simulink model "InvertedPendulumSSTest"  (Simulink 7.7)
settings: Solver=ode5  StartTime=0.0  StopTime=10  FixedStep=.0005  RelTol=1e-3
PreLoadFcn:
  | StateSpacePrelimv2
values from neighbouring files (symbols this model uses):
  ba = 6.5E-6    (= 6.5e-06)    [StateSpacePrelimv2.m]
  btf = 1.08586e-5    (= 1.08586e-05)    [StateSpacePrelimv2.m]
  btr = 4.8593e-5    (= 4.8593e-05)    [StateSpacePrelimv2.m]
  CONTROLLER_SWITCH_POINT = .30    (= 0.3)    [StateSpacePrelimv2.m]
  g = 9.81    [StateSpacePrelimv2.m]
  I1zt = 6.78e-4 + 3.50514e-5    (= 0.0007130514)    [StateSpacePrelimv2.m]
  Ix2 = 8.1e-6    (= 8.1e-06)    [StateSpacePrelimv2.m]
  Ixz2 = 2.03e-5    (= 2.03e-05)    [StateSpacePrelimv2.m]
  Iy2 = 3.711e-4    (= 0.0003711)    [StateSpacePrelimv2.m]
  Iz2 = 3.646e-4    (= 0.0003646)    [StateSpacePrelimv2.m]
  K = lqr(A,B,Q,R)    [StateSpacePrelimv2.m]
  Ka = 1    [StateSpacePrelimv2.m]
  Kb = 0.04    [StateSpacePrelimv2.m]
  Kt = 0.0314499    [StateSpacePrelimv2.m]
  l1 = 0.10825640    (= 0.1082564)    [StateSpacePrelimv2.m]
  l2c = 0.0856786    [StateSpacePrelimv2.m]
  m2 = 0.0820142    [StateSpacePrelimv2.m]
  Rm = 1.85    [StateSpacePrelimv2.m]
  tau = .01    (= 0.01)    [StateSpacePrelimv2.m]
  Tca = 7e-6    (= 7e-06)    [StateSpacePrelimv2.m]
  Tctf = 0.022439    [StateSpacePrelimv2.m]
  Tctr = 0.0143096    [StateSpacePrelimv2.m]
  Vsupply = 24    [StateSpacePrelimv2.m]
settings Model: Creator=gshiva  LastModifiedBy=jrpeterson

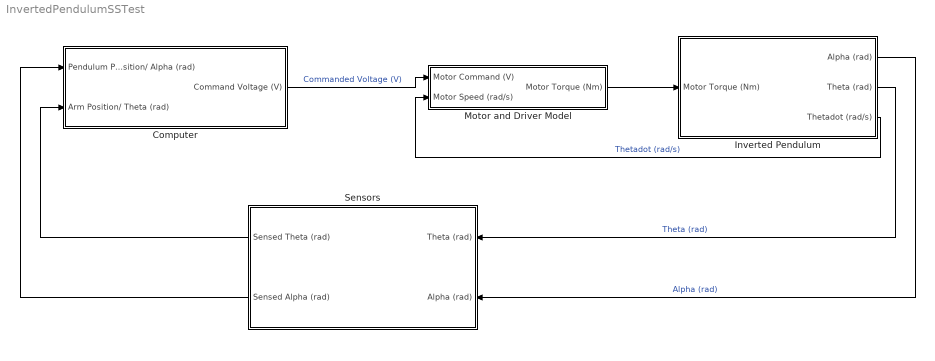
== system InvertedPendulumSSTest ==
  Computer : Subsystem
  Inverted Pendulum : Subsystem
  Motor and Driver Model : Subsystem
  Sensors : Subsystem
  wires:
  Computer/1(Command Voltage (V)) -> Motor and Driver Model/1(Motor Command (V))  "Commanded Voltage (V)"
  Sensors/2(Sensed Alpha (rad)) -> Computer/1(Pendulum Position/ Alpha (rad))
  Sensors/1(Sensed Theta (rad)) -> Computer/2(Arm Position/ Theta (rad))
  Inverted Pendulum/2(Theta (rad)) -> Sensors/1(Theta (rad))  "Theta (rad)"
  Inverted Pendulum/1(Alpha (rad)) -> Sensors/2(Alpha (rad))  "Alpha (rad)"
  Motor and Driver Model/1(Motor Torque (Nm)) -> Inverted Pendulum/1(Motor Torque (Nm))
  Inverted Pendulum/3(Thetadot (rad/s)) -> Motor and Driver Model/2(Motor Speed (rad/s))  "Thetadot (rad/s)"

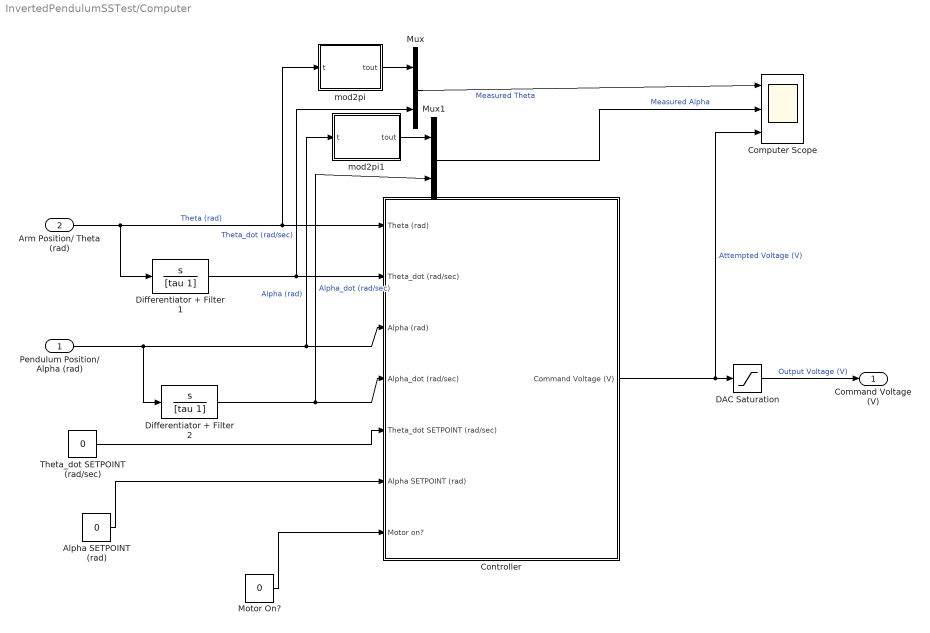
== system InvertedPendulumSSTest/Computer ==
  Pendulum Position/ Alpha (rad) : Inport
  Arm Position/ Theta (rad) : Inport  Port=2
  Alpha SETPOINT (rad) : Constant  Value=0
  Computer Scope : Scope  NumInputPorts=3
      settings: YMin=-10~-25~-800000  YMax=17.5~325~900000  SaveName=ScopeData3
  Controller : Subsystem
  DAC Saturation : Saturate  UpperLimit=10  LowerLimit=-10
  Differentiator + Filter 1 : TransferFcn  Numerator=[1 0]  Denominator=[tau 1]
  Differentiator + Filter 2 : TransferFcn  Numerator=[1 0]  Denominator=[tau 1]
  Motor On? : Constant  Value=0
  Mux : Mux  Inputs=2
  Mux1 : Mux  Inputs=2
  Theta_dot SETPOINT (rad/sec) : Constant  Value=0
  mod2pi : Stateflow chart  TreatAsAtomicUnit=on
  mod2pi1 : Stateflow chart  TreatAsAtomicUnit=on
  Command Voltage (V) : Outport
  wires:
  DAC Saturation/1 -> Command Voltage (V)/1  "Output Voltage (V)"
  Arm Position/ Theta (rad)/1 -> Differentiator + Filter 1/1, Controller/1(Theta (rad)), mod2pi/1(t)  "Theta (rad)"
  Differentiator + Filter 1/1 -> Controller/2(Theta_dot (rad/sec)), Mux/2  "Theta_dot (rad/sec)"
  Pendulum Position/ Alpha (rad)/1 -> Differentiator + Filter 2/1, Controller/3(Alpha (rad)), mod2pi1/1(t)  "Alpha (rad)"
  Differentiator + Filter 2/1 -> Mux1/2, Controller/4(Alpha_dot (rad/sec))  "Alpha_dot (rad/sec)"
  Controller/1(Command Voltage (V)) -> DAC Saturation/1, Computer Scope/3  "Attempted Voltage (V)"
  Theta_dot SETPOINT (rad/sec)/1 -> Controller/5(Theta_dot SETPOINT (rad/sec))
  Alpha SETPOINT (rad)/1 -> Controller/6(Alpha SETPOINT (rad))
  Mux/1 -> Computer Scope/1  "Measured Theta"
  Mux1/1 -> Computer Scope/2  "Measured Alpha"
  Motor On?/1 -> Controller/7(Motor on?)
  mod2pi/1(tout) -> Mux/1
  mod2pi1/1(tout) -> Mux1/1

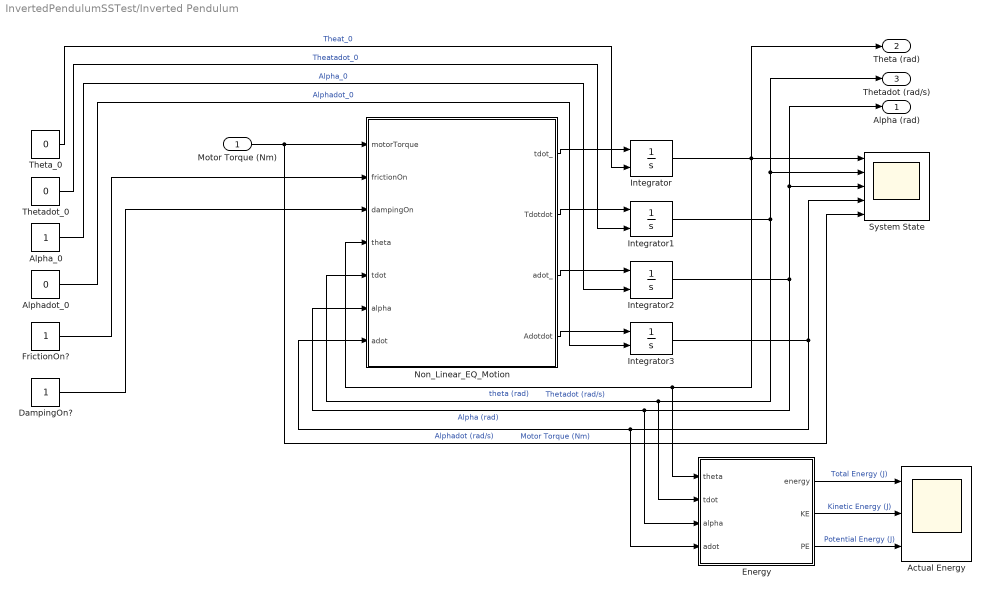
== system InvertedPendulumSSTest/Inverted Pendulum ==
  Motor Torque (Nm) : Inport
  Actual Energy : Scope  NumInputPorts=3
      settings: TimeRange=5  YMin=-0.07~0~-0.14  YMax=0.1~0.175~1.38778e-17  SaveName=Actual_Energy
  Alpha_0 : Constant
  Alphadot_0 : Constant  Value=0
  DampingOn? : Constant
  Energy : Stateflow chart  TreatAsAtomicUnit=on
  FrictionOn? : Constant
  Integrator{,1..3} (4 alike) : Integrator  InitialConditionSource=external
  Non_Linear_EQ_Motion : Stateflow chart  TreatAsAtomicUnit=on
  System State : Scope  NumInputPorts=5
      settings: TimeRange=10  YMin=-1~-20~0~-20~-0.4  YMax=4~20~5~20~0.4
  Theta_0 : Constant  Value=0
  Thetadot_0 : Constant  Value=0
  Alpha (rad) : Outport
  Theta (rad) : Outport  Port=2
  Thetadot (rad/s) : Outport  Port=3
  wires:
  Motor Torque (Nm)/1 -> Non_Linear_EQ_Motion/1(motorTorque), System State/5  "Motor Torque (Nm)"
  Non_Linear_EQ_Motion/1(tdot_) -> Integrator/1
  Theta_0/1 -> Integrator/2  "Theat_0"
  Non_Linear_EQ_Motion/2(Tdotdot) -> Integrator1/1
  Non_Linear_EQ_Motion/3(adot_) -> Integrator2/1
  Non_Linear_EQ_Motion/4(Adotdot) -> Integrator3/1
  Thetadot_0/1 -> Integrator1/2  "Theatadot_0"
  Alpha_0/1 -> Integrator2/2  "Alpha_0"
  Alphadot_0/1 -> Integrator3/2  "Alphadot_0"
  Integrator/1 -> System State/1, Theta (rad)/1, Non_Linear_EQ_Motion/4(theta), Energy/1(theta)  "theta (rad)"
  Integrator1/1 -> Non_Linear_EQ_Motion/5(tdot), Energy/2(tdot), System State/2, Thetadot (rad/s)/1  "Thetadot (rad/s)"
  Integrator2/1 -> System State/3, Alpha (rad)/1, Non_Linear_EQ_Motion/6(alpha), Energy/3(alpha)  "Alpha (rad)"
  Integrator3/1 -> System State/4, Non_Linear_EQ_Motion/7(adot), Energy/4(adot)  "Alphadot (rad/s)"
  Energy/1(energy) -> Actual Energy/1  "Total Energy (J)"
  Energy/2(KE) -> Actual Energy/2  "Kinetic Energy (J)"
  Energy/3(PE) -> Actual Energy/3  "Potential Energy (J)"
  FrictionOn?/1 -> Non_Linear_EQ_Motion/2(frictionOn)
  DampingOn?/1 -> Non_Linear_EQ_Motion/3(dampingOn)

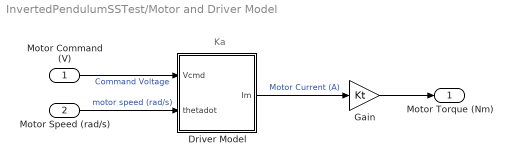
== system InvertedPendulumSSTest/Motor and Driver Model ==
  note: Ka
  Motor Command (V) : Inport
  Motor Speed (rad/s) : Inport  Port=2
  Driver Model : Stateflow chart  TreatAsAtomicUnit=on
  Gain : Gain  Gain=Kt
  Motor Torque (Nm) : Outport
  wires:
  Gain/1 -> Motor Torque (Nm)/1
  Driver Model/1(Im) -> Gain/1  "Motor Current (A)"
  Motor Command (V)/1 -> Driver Model/1(Vcmd)  "Command Voltage"
  Motor Speed (rad/s)/1 -> Driver Model/2(thetadot)  "motor speed (rad/s)"

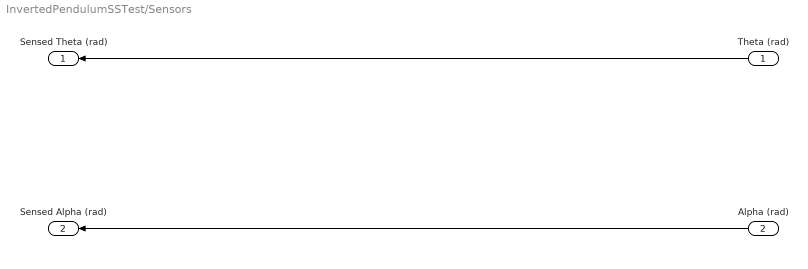
== system InvertedPendulumSSTest/Sensors ==
  Theta (rad) : Inport
  Alpha (rad) : Inport  Port=2
  Sensed Theta (rad) : Outport
  Sensed Alpha (rad) : Outport  Port=2
  wires:
  Alpha (rad)/1 -> Sensed Alpha (rad)/1
  Theta (rad)/1 -> Sensed Theta (rad)/1

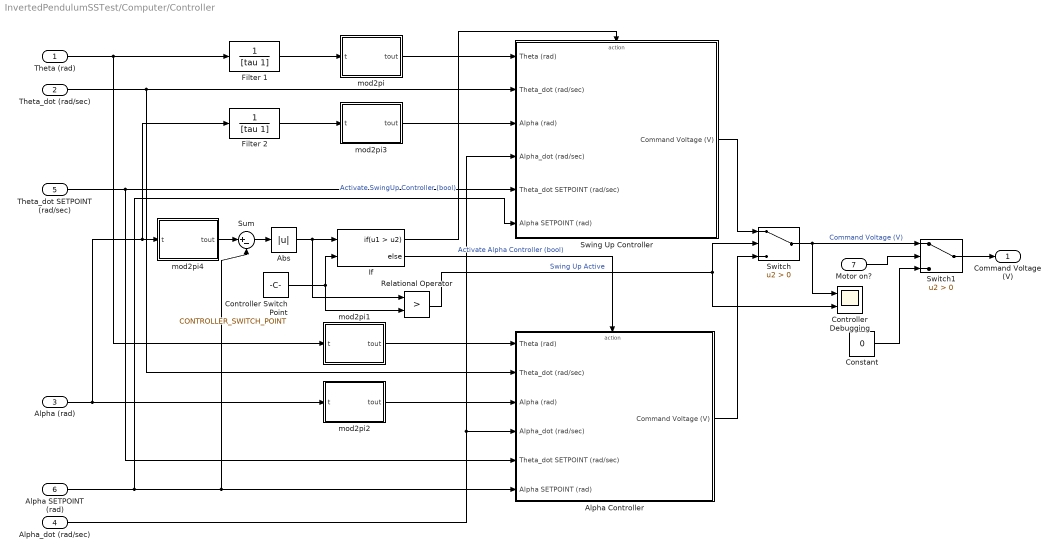
== system InvertedPendulumSSTest/Computer/Controller ==
  Theta (rad) : Inport
  Theta_dot (rad/sec) : Inport  Port=2
  Alpha (rad) : Inport  Port=3
  Alpha_dot (rad/sec) : Inport  Port=4
  Theta_dot SETPOINT (rad/sec) : Inport  Port=5
  Alpha SETPOINT (rad) : Inport  Port=6
  Motor on? : Inport  Port=7
  Abs : Abs
  Alpha Controller : Subsystem  TreatAsAtomicUnit=on
  Constant : Constant  Value=0
  Controller Debugging : Scope  NumInputPorts=2
      settings: YMin=-5~-5  YMax=5~5  SaveName=ScopeData2
  Controller Switch Point : Constant  Value=CONTROLLER_SWITCH_POINT
  Filter 1 : TransferFcn  Denominator=[tau 1]
  Filter 2 : TransferFcn  Denominator=[tau 1]
  If : If  NumInputs=2  IfExpression=u1 > u2
  Relational Operator : RelationalOperator  Operator=>  OutDataTypeStr=boolean
  Sum : Sum  Inputs=|+-
  Swing Up Controller : Subsystem  TreatAsAtomicUnit=on
  Switch : Switch  Criteria=u2 > Threshold
  Switch1 : Switch  Criteria=u2 > Threshold
  mod2pi : Stateflow chart  TreatAsAtomicUnit=on
  mod2pi1 : Stateflow chart  TreatAsAtomicUnit=on
  mod2pi2 : Stateflow chart  TreatAsAtomicUnit=on
  mod2pi3 : Stateflow chart  TreatAsAtomicUnit=on
  mod2pi4 : Stateflow chart  TreatAsAtomicUnit=on
  Command Voltage (V) : Outport
  wires:
  If/2 -> Alpha Controller/Action  "Activate Alpha Controller (bool)"
  Switch/1 -> Controller Debugging/1, Switch1/1  "Command Voltage (V)"
  If/1 -> Swing Up Controller/Action  "Activate SwingUp Controller (bool)"
  Controller Switch Point/1 -> If/2, Relational Operator/2
  Sum/1 -> Abs/1
  Alpha SETPOINT (rad)/1 -> Swing Up Controller/6(Alpha SETPOINT (rad)), Sum/2, Alpha Controller/6(Alpha SETPOINT (rad))
  Theta (rad)/1 -> mod2pi1/1(t), Filter 1/1
  Theta_dot (rad/sec)/1 -> Swing Up Controller/2(Theta_dot (rad/sec)), Alpha Controller/2(Theta_dot (rad/sec))
  Theta_dot SETPOINT (rad/sec)/1 -> Swing Up Controller/5(Theta_dot SETPOINT (rad/sec)), Alpha Controller/5(Theta_dot SETPOINT (rad/sec))
  Alpha_dot (rad/sec)/1 -> Swing Up Controller/4(Alpha_dot (rad/sec)), Alpha Controller/4(Alpha_dot (rad/sec))
  Alpha (rad)/1 -> Filter 2/1, mod2pi4/1(t), mod2pi2/1(t)
  Swing Up Controller/1(Command Voltage (V)) -> Switch/1
  Alpha Controller/1(Command Voltage (V)) -> Switch/3
  Relational Operator/1 -> Switch/2, Controller Debugging/2  "Swing Up Active"
  Switch1/1 -> Command Voltage (V)/1
  Constant/1 -> Switch1/3
  Motor on?/1 -> Switch1/2
  mod2pi/1(tout) -> Swing Up Controller/1(Theta (rad))
  mod2pi1/1(tout) -> Alpha Controller/1(Theta (rad))
  mod2pi2/1(tout) -> Alpha Controller/3(Alpha (rad))
  mod2pi3/1(tout) -> Swing Up Controller/3(Alpha (rad))
  Filter 1/1 -> mod2pi/1(t)
  Filter 2/1 -> mod2pi3/1(t)
  Abs/1 -> If/1, Relational Operator/1
  mod2pi4/1(tout) -> Sum/1

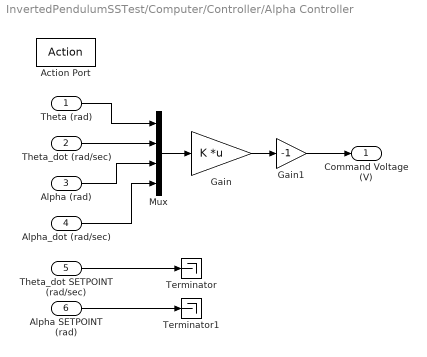
== system InvertedPendulumSSTest/Computer/Controller/Alpha Controller ==
  Theta (rad) : Inport
  Theta_dot (rad/sec) : Inport  Port=2
  Alpha (rad) : Inport  Port=3
  Alpha_dot (rad/sec) : Inport  Port=4
  Theta_dot SETPOINT (rad/sec) : Inport  Port=5
  Alpha SETPOINT (rad) : Inport  Port=6
  Action Port : ActionPort  ActionType=else
  Gain : Gain  Gain=K  Multiplication=Matrix(K*u)
  Gain1 : Gain  Gain=-1
  Mux : Mux
  Terminator : Terminator
  Terminator1 : Terminator
  Command Voltage (V) : Outport
  wires:
  Theta (rad)/1 -> Mux/1
  Theta_dot (rad/sec)/1 -> Mux/2
  Alpha (rad)/1 -> Mux/3
  Alpha_dot (rad/sec)/1 -> Mux/4
  Mux/1 -> Gain/1
  Gain/1 -> Gain1/1
  Gain1/1 -> Command Voltage (V)/1
  Theta_dot SETPOINT (rad/sec)/1 -> Terminator/1
  Alpha SETPOINT (rad)/1 -> Terminator1/1

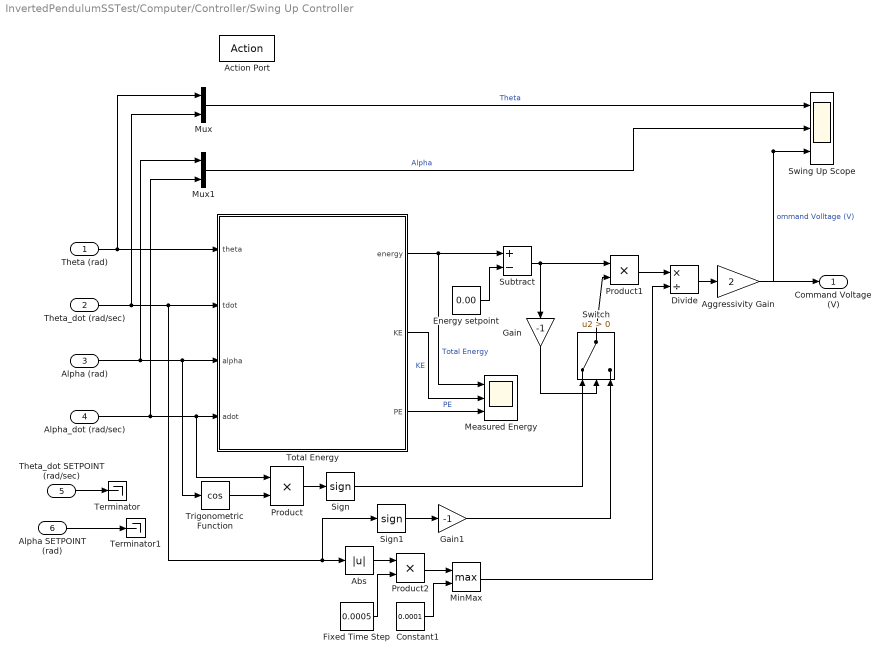
== system InvertedPendulumSSTest/Computer/Controller/Swing Up Controller ==
  Theta (rad) : Inport
  Theta_dot (rad/sec) : Inport  Port=2
  Alpha (rad) : Inport  Port=3
  Alpha_dot (rad/sec) : Inport  Port=4
  Theta_dot SETPOINT (rad/sec) : Inport  Port=5
  Alpha SETPOINT (rad) : Inport  Port=6
  Action Port : ActionPort  ActionType=then
  Abs : Abs
  Aggressivity Gain : Gain  Gain=2
  Constant1 : Constant  Value=0.0001
  Divide : Product  Inputs=*/
  Energy setpoint : Constant  Value=0.00
  Fixed Time Step : Constant  Value=0.0005
  Gain : Gain  Gain=-1
  Gain1 : Gain  Gain=-1
  Measured Energy : Scope  NumInputPorts=3
      settings: TimeRange=10  YMin=-0.065~0~-0.14  YMax=-0.035~0.1~-0.02000000000000002  SaveName=Measured_Energy
  MinMax : MinMax  Function=max  Inputs=2
  Mux : Mux  Inputs=2
  Mux1 : Mux  Inputs=2
  Product : Product  RndMeth=Zero
  Product1 : Product  RndMeth=Zero
  Product2 : Product  RndMeth=Zero
  Sign : Signum
  Sign1 : Signum
  Subtract : Sum  Inputs=+-
  Swing Up Scope : Scope  NumInputPorts=3
      settings: TimeRange=5  YMin=-15~-4~-15  YMax=5~4~15  SaveName=ScopeData4
  Switch : Switch  Criteria=u2 > Threshold
  Terminator : Terminator
  Terminator1 : Terminator
  Total Energy : Stateflow chart  TreatAsAtomicUnit=on
  Trigonometric Function : Trigonometry  Operator=cos
  Command Voltage (V) : Outport
  wires:
  Theta (rad)/1 -> Total Energy/1(theta), Mux/1
  Theta_dot (rad/sec)/1 -> Mux/2, Total Energy/2(tdot), Abs/1, Sign1/1
  Alpha (rad)/1 -> Total Energy/3(alpha), Trigonometric Function/1, Mux1/1
  Alpha_dot (rad/sec)/1 -> Total Energy/4(adot), Product/1, Mux1/2
  Trigonometric Function/1 -> Product/2
  Product/1 -> Sign/1
  Subtract/1 -> Product1/1, Gain/1
  Total Energy/2(KE) -> Measured Energy/2  "KE"
  Aggressivity Gain/1 -> Swing Up Scope/3, Command Voltage (V)/1  "ommand Volltage (V)"
  Theta_dot SETPOINT (rad/sec)/1 -> Terminator/1
  Alpha SETPOINT (rad)/1 -> Terminator1/1
  Mux1/1 -> Swing Up Scope/2  "Alpha"
  Mux/1 -> Swing Up Scope/1  "Theta"
  Total Energy/3(PE) -> Measured Energy/3  "PE"
  Abs/1 -> Product2/1
  Fixed Time Step/1 -> Product2/2
  Product2/1 -> MinMax/1
  Constant1/1 -> MinMax/2
  Product1/1 -> Divide/1
  Divide/1 -> Aggressivity Gain/1
  Energy setpoint/1 -> Subtract/2
  Total Energy/1(energy) -> Subtract/1, Measured Energy/1  "Total Energy"
  Sign/1 -> Switch/1
  Switch/1 -> Product1/2
  Gain1/1 -> Switch/3
  Gain/1 -> Switch/2
  Sign1/1 -> Gain1/1
  MinMax/1 -> Divide/2

== matlab function Inverted Pendulum/Energy ==
  data: theta input double; energy output double; tdot input double; alpha input double; adot input double; Iz2 parameter double; l2c parameter double; Iy2 parameter double; l1 parameter double; Ixz2 parameter double; I1zt parameter double; Ix2 parameter double; m2 parameter double; g parameter double; KE output double; PE output double
function [energy, KE, PE]  = totalEnergy(theta, tdot, alpha, adot, Iz2,l2c,Iy2,l1,Ixz2,I1zt,Ix2,m2,g)

% Iz2 = 3.646e-4;
% l2c = 0.0856786;
% Iy2 = 3.711e-4;
% l1 = 0.1016;
% Ixz2 = 2.03e-5;
% I1zt = 6.78e-4;
% Ix2 = 8.1e-6;
% m2 = 0.0820142;
% g = 9.81;

%%%%%%%%%%%%%%%%%%%%%%%%%%%%%%%%%%%%%%%%%%%%%%%%%%%%%%%%%%%%%%%%%%%%%%%%%%%
% compute potential energy of the system only cares about the pendulum
ca = cos(alpha); sa = sin(alpha);
ct = cos(theta); st = sin(theta);

PE = (ca - 1)*l2c*m2*g;
%%%%%%%%%%%%%%%%%%%%%%%%%%%%%%%%%%%%%%%%%%%%%%%%%%%%%%%%%%%%%%%%%%%%%%%%%%%

% compute the kinetic energy of the the system
thetadot = tdot;  alphadot = adot;

% rotational component for arm
KE1 = 0.5*I1zt*thetadot*thetadot;

%%%%%%%%%%%%%%%%%%%%%%%%%%%%%%%%%%%%%%%%%%%%%%%%%%
% translational component for pendulum
J = zeros(3,2);

J(1,1) = -l2c*sa*ct - l1*st;
J(1,2) = -l2c*st*ca;

J(2,1) = -l2c*sa*st + l1*ct;
J(2,2) = l2c*ct*ca;

J(3,2) = -l2c*sa;

% now that we have the jacobian
V = J*[thetadot; alphadot];

%%%%%%%%%%%%%%%%%%%%%%%%%%%%%%%%%%%%%%%%%%%%%%%%%%
KE2T = 0.5*m2*(V'*V);

% rotaional component
KE2R = 0.5*(thetadot*thetadot*(Ix2*ca*ca + Iy2*sa*sa) - 2*Ixz2*thetadot*alphadot*ca ...
    + Iz2*alphadot*alphadot);

KE = KE1 + KE2T + KE2R;

energy = KE + PE;

== matlab function Inverted Pendulum/Non_Linear_EQ_Motion ==
  data: motorTorque input double; frictionOn input double; dampingOn input double; theta input double; tdot_ output double; tdot input double; alpha input double; adot input double; Tdotdot output double; adot_ output double; Adotdot output double; Iz2 parameter double; l2c parameter double; Iy2 parameter double; l1 parameter double; Ixz2 parameter double; I1zt parameter double; Ix2 parameter double; m2 parameter double; g parameter double; ba parameter double; btf parameter double; btr parameter double; Tca parameter double; Tctf parameter double; Tctr parameter double
function [tdot_, Tdotdot, adot_, Adotdot]  = eqMotionLagrange(motorTorque, frictionOn , dampingOn ,theta, tdot, alpha, adot, Iz2,l2c,Iy2,l1,Ixz2,I1zt,Ix2,m2,g,ba,btf,btr,Tca,Tctf,Tctr)
% we currently assume differential coulomb friction and damping for theta,
% but not for alpha
%global m2 I1zt Ix2 Iy2 Iz2 Ixz2 g l1 l2c ba btf btr

% Iz2 = 3.646e-4;
% l2c = 0.0856786;
% Iy2 = 3.711e-4;
% l1 = 0.1016;
% Ixz2 = 2.03e-5;
% I1zt = 6.78e-4;
% Ix2 = 8.1e-6;
% m2 = 0.0820142;
% g = 9.81; ba = 6.5E-6; btf = 1.08586e-5; btr = 4.8593e-5;
% %Tca = 7e-6; Tctf = 0.022439; Tctr = 0.0143096; 
% Tca = 7e-6; Tctf = 0.00; Tctr = 0.00; 

% theta = x(1); tdot = x(2); ct = cos(theta); st = sin(theta);
% alpha = x(3); adot = x(4); ca = cos(alpha); sa = sin(alpha);
tdot_ = tdot;
adot_ = adot;
%ct = cos(theta); st = sin(theta);
ca = cos(alpha); sa = sin(alpha);
%%%%%%%%%%%
% Motor
Tm = motorTorque;  % placeholder for motor power term

%%%%%%%%%%%%
% Damping
% model damping differently forwards and backwards for theta
if dampingOn
    if (tdot > 0)
        Bt = btf;  % baf opposes forwards motion for theta
    elseif (tdot < 0)
        Bt = btr; % bar opposes reverse motion for theta
    else
        Bt = 0;
    end
    Ba = ba;
else
    Bt = 0;
    Ba = 0;
end
% for alpha only a single viscous damping term

%%%%%%%%%%%%%%
% Friction
if frictionOn
    TCt = coulombFriction(Tctf, Tctr, Tm, tdot);
    Tg = m2*g*l2c*sa; % torque exerted by gravity on pendulum
    TCa = coulombFriction(Tca, Tca, Tg, adot);
else 
    TCa = 0;
    TCt = 0;
end


C1 = Iz2+m2*l2c*l2c;  C2 = Iy2+m2*l2c*l2c;   C3 = m2*l1*l2c-Ixz2;  C4 = l2c*m2*g;

D = (I1zt + sa*sa*C2 + Ix2*ca*ca + m2*l1*l1)*C1 - ca*ca*C3*C3;

Tdotdot = (1/D)*(-2*tdot*adot*sa*ca*(C2-Ix2)*C1 + adot*adot*sa*C3*C1 ...
    - tdot*tdot*sa*ca*ca*(C2-Ix2)*C3 + adot*Ba*ca*C3 - sa*ca*C3*C4 - TCa*ca*C3 ...
    - Bt*tdot*C1 + Tm*C1 + TCt*C1);

Adotdot = (1/C1)*(-Tdotdot*ca*C3 + tdot*tdot*sa*ca*(C2-Ix2) + C4*sa - Ba*adot + TCa);

end
% xdot = [tdot; Tdotdot; adot; Adotdot];

%-------------------------------------------------
function [torque] = coulombFriction(Tff, Tfr, externalTorque, thetadot)
% this friction model is making an assumption that isn't strictly true, we
% have static friction, but only the external torque exerted on each link
% will be considered.  This is not strictly correct, really we should
% consider the constraint forces as well
% it might not hold with the strength that it should

staticThreshold = 1e-6;
staticRatio = 1;

if (abs(thetadot) < staticThreshold) % if not moving, friction opposes attempted motion
    % if external torque does not exceed static friction
    if ((externalTorque < Tff) && (externalTorque >= 0)) || ((externalTorque > -Tfr) && (externalTorque < 0))
        FF = abs(externalTorque);
    elseif (externalTorque > Tff)
        FF = Tff;
    else
        FF = Tfr;
    end
    torque = - staticRatio * FF * sign(externalTorque);
    
else % if we are moving oppose the actual motion with kinetic friciton
    if thetadot > staticThreshold
        torque = -Tff;
    else
        torque = Tfr;
    end
end
end
%------------------------------------------------

== matlab function Computer/Controller/Swing Up Controller/Total Energy ==
  data: theta input double; energy output double; tdot input double; alpha input double; adot input double; Iz2 parameter double; l2c parameter double; Iy2 parameter double; l1 parameter double; Ixz2 parameter double; I1zt parameter double; Ix2 parameter double; m2 parameter double; g parameter double; KE output double; PE output double
function [energy, KE, PE]  = totalEnergy(theta, tdot, alpha, adot, Iz2,l2c,Iy2,l1,Ixz2,I1zt,Ix2,m2,g)

% Iz2 = 3.646e-4;
% l2c = 0.0856786;
% Iy2 = 3.711e-4;
% l1 = 0.1016;
% Ixz2 = 2.03e-5;
% I1zt = 6.78e-4;
% Ix2 = 8.1e-6;
% m2 = 0.0820142;
% g = 9.81;

%%%%%%%%%%%%%%%%%%%%%%%%%%%%%%%%%%%%%%%%%%%%%%%%%%%%%%%%%%%%%%%%%%%%%%%%%%%
% compute potential energy of the system only cares about the pendulum
ca = cos(alpha); sa = sin(alpha);
ct = cos(theta); st = sin(theta);

PE = (ca - 1)*l2c*m2*g;
%%%%%%%%%%%%%%%%%%%%%%%%%%%%%%%%%%%%%%%%%%%%%%%%%%%%%%%%%%%%%%%%%%%%%%%%%%%

% compute the kinetic energy of the the system
thetadot = tdot;  alphadot = adot;

% rotational component for arm
KE1 = 0.5*I1zt*thetadot*thetadot;

%%%%%%%%%%%%%%%%%%%%%%%%%%%%%%%%%%%%%%%%%%%%%%%%%%
% translational component for pendulum
J = zeros(3,2);

J(1,1) = -l2c*sa*ct - l1*st;
J(1,2) = -l2c*st*ca;

J(2,1) = -l2c*sa*st + l1*ct;
J(2,2) = l2c*ct*ca;

J(3,2) = -l2c*sa;

% now that we have the jacobian
V = J*[thetadot; alphadot];

%%%%%%%%%%%%%%%%%%%%%%%%%%%%%%%%%%%%%%%%%%%%%%%%%%
KE2T = 0.5*m2*(V'*V);

% rotaional component
KE2R = 0.5*(thetadot*thetadot*(Ix2*ca*ca + Iy2*sa*sa) - 2*Ixz2*thetadot*alphadot*ca ...
    + Iz2*alphadot*alphadot);

KE = KE1+KE2T+KE2R;% neglecting energy of swing arm

energy = KE + PE;

== matlab function Motor and Driver Model/Driver Model ==
  data: Vcmd input double; Im output double; Vsupply parameter double; thetadot input double; Kb parameter double; Ka parameter double; Rm parameter double
function Im = fcn(Vcmd, Vsupply, thetadot, Kb, Ka, Rm)
% determines motor current as a function of the command voltage, supply
% voltages, angular speed, and motor back emf constant
% Vsupply are the supplied votages to the power supply
% thetadot is the current angular speed of the motor
% Kb is the back emf constant
% Ka is the nominal motor driver gain
% R is nominanal motor resistance

% for thetadot no load = 600 rad/s then Kb = 0.04

% for the given command current, how much voltage would we need
Vb = Kb*thetadot;
Icmd = Ka * Vcmd;
Vrequired = Vb + Rm * Icmd;

if abs(Vrequired) < Vsupply
    Im = Icmd; % if we can supply enough voltage, then we can send this much current
else
    % otherwise, need to figure out what current we are limited to
    if Vcmd > 0
        Im = (Vsupply - Vb) / Rm;
    else
        Im = (-Vsupply - Vb) / Rm;
    end
end
end

== matlab function Computer/Controller/mod2pi1 ==
  data: t input double; tout output double
function tout = mod2pi(t)
% returns an angle between pi and -pi

if t < 0
    tout = -mod2pi_sub(-t);
else
    tout = mod2pi_sub(t);
end
end

function [tout] = mod2pi_sub(t)
% only good for positive numbers
tout = t - floor(t*0.5/pi + 0.5) * 2*pi;
end

== matlab function Computer/Controller/mod2pi2 ==
  data: t input double; tout output double
function tout = mod2pi(t)
% returns an angle between pi and -pi

if t < 0
    tout = -mod2pi_sub(-t);
else
    tout = mod2pi_sub(t);
end
end

function [tout] = mod2pi_sub(t)
% only good for positive numbers
tout = t - floor(t*0.5/pi + 0.5) * 2*pi;
end

== matlab function Computer/Controller/mod2pi ==
  data: t input double; tout output double
function tout = mod2pi(t)
% returns an angle between pi and -pi

if t < 0
    tout = -mod2pi_sub(-t);
else
    tout = mod2pi_sub(t);
end
end

function [tout] = mod2pi_sub(t)
% only good for positive numbers
tout = t - floor(t*0.5/pi + 0.5) * 2*pi;
end

== matlab function Computer/mod2pi ==
  data: t input double; tout output double
function tout = mod2pi(t)
% returns an angle between pi and -pi

if t < 0
    tout = -mod2pi_sub(-t);
else
    tout = mod2pi_sub(t);
end
end

function [tout] = mod2pi_sub(t)
% only good for positive numbers
tout = t - floor(t*0.5/pi + 0.5) * 2*pi;
end

== matlab function Computer/Controller/mod2pi3 ==
  data: t input double; tout output double
function tout = mod2pi(t)
% returns an angle between pi and -pi

if t < 0
    tout = -mod2pi_sub(-t);
else
    tout = mod2pi_sub(t);
end
end

function [tout] = mod2pi_sub(t)
% only good for positive numbers
tout = t - floor(t*0.5/pi + 0.5) * 2*pi;
end

== matlab function Computer/mod2pi1 ==
  data: t input double; tout output double
function tout = mod2pi(t)
% returns an angle between pi and -pi

if t < 0
    tout = -mod2pi_sub(-t);
else
    tout = mod2pi_sub(t);
end
end

function [tout] = mod2pi_sub(t)
% only good for positive numbers
tout = t - floor(t*0.5/pi + 0.5) * 2*pi;
end

== matlab function Computer/Controller/mod2pi4 ==
  data: t input double; tout output double
function tout = mod2pi(t)
% returns an angle between pi and -pi

if t < 0
    tout = -mod2pi_sub(-t);
else
    tout = mod2pi_sub(t);
end
end

function [tout] = mod2pi_sub(t)
% only good for positive numbers
tout = t - floor(t*0.5/pi + 0.5) * 2*pi;
end
